simulink model "mass_spring_damper_animation"  (R2015a)
settings: Solver=ode45  StartTime=0.0  StopTime=inf  RelTol=1e-3
undefined symbols (not defined in the file): drawMassSpringDamper
libraries: simulink x1
settings Model: Creator=ecestudent  LastModifiedBy=ecestudent

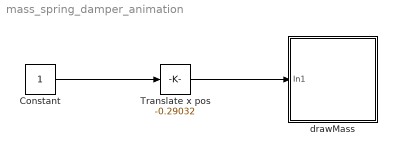
== system mass_spring_damper_animation ==
  Constant : Constant
  Translate x pos : simulink/Math Operations/Slider Gain  low=-1  gain=-0.29032  high=1
  drawMass : Subsystem
      mask Display: image(imread('tv.jpg'))
  wires:
  Constant/1 -> Translate x pos/1
  Translate x pos/1 -> drawMass/1(In1)

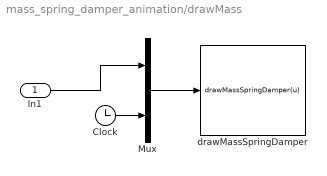
== system mass_spring_damper_animation/drawMass ==
  In1 : Inport
  Clock : Clock
  Mux : Mux  Inputs=2
  drawMassSpringDamper : MATLABFcn  MATLABFcn=drawMassSpringDamper(u)  OutputDimensions=0
      mask Display: image(imread('tv.jpg'))
  wires:
  In1/1 -> Mux/1
  Clock/1 -> Mux/2
  Mux/1 -> drawMassSpringDamper/1
